simulink model "PassStFwdbkwdHolderChk"  (R2018b)
settings: Solver=FixedStepDiscrete  StartTime=0.0  StopTime=10.0  RelTol=1e-3
libraries: simulink x1
settings Model: Creator=sn2xws  LastModifiedBy=sn2xws
settings Model: ModifiedHistory=|
  | 2024.6.26 V3.0.0 557模式流程
  | 2024.11.18 V3.0.1 增加Md58 Retry
  | 2024.12.11 V3.0.2 Md57 Md58 反复retry的bug修复 BUG 960388 BUG 960408
  | 25.7.4 V3.13.0 新增Md61 Md62
settings DataIOCC: SaveFormat=StructureWithTime
settings OptimizationCC: DefaultParameterBehavior=Inlined  EnhancedBackFolding=on  PassReuseOutputArgsAs=Individual arguments  ZeroExternalMemoryAtStartup=off  ZeroInternalMemoryAtStartup=off  OptimizeBlockOrder=speed  DifferentSizesBufferReuse=on  OptimizationCustomize=off
settings DebuggingCC: ParameterTunabilityLossMsg=error
settings SFSimCC: MATLABDynamicMemAlloc=off
settings RTWCC: SystemTargetFile=autosar.tlc  GenCodeOnly=on  TemplateMakefile=ert_default_tmf  Description=AUTOSAR  GenerateReport=on  IncludeHyperlinkInReport=on  LaunchReport=on  GenerateTraceInfo=on  GenerateTraceReport=on  GenerateTraceReportSl=on  GenerateTraceReportSf=on  GenerateTraceReportEml=on
settings CodeAppCC: ForceParamTrailComments=on  IgnoreCustomStorageClasses=off  OperatorAnnotations=on  SimulinkDataObjDesc=on  SFDataObjDesc=on  InsertBlockDesc=on
settings STFCustomTargetCC: TargetLangStandard=C99 (ISO)  MultiwordLength=256  ParMdlRefBuildCompliant=on  CompOptLevelCompliant=on  IncludeMdlTerminateFcn=off  CombineOutputUpdateFcns=on  SuppressErrorStatus=on  ERTCustomFileBanners=on  SupportNonFinite=off  SupportComplex=off  SupportContinuousTime=off  SupportNonInlinedSFcns=off  RemoveResetFunc=on  MATLABClassNameForMDSCustomization=Simulink.SoftwareTarget.ERTCustomization  AutosarCompliant=on  UseToolchainInfoCompliant=on  LookupTableObjectStructAxisOrder=2,1,3,4,...  LUTObjectStructOrderEvenSpacing=Size,Table,Breakpoints  SystemTargetFile=autosar.tlc
settings ERTTargetCC: TargetLangStandard=C99 (ISO)  ConcurrentExecutionCompliant=off  IncludeMdlTerminateFcn=off  SuppressErrorStatus=on  SupportNonFinite=off  SupportComplex=off  ModelStepFunctionPrototypeControlCompliant=off  CPPClassGenCompliant=off  AutosarCompliant=on  LookupTableObjectStructAxisOrder=2,1,3,4,...  LUTObjectStructOrderEvenSpacing=Size,Table,Breakpoints  InlinedParameterPlacement=NonHierarchical  ERTCustomFileTemplate=example_file_process.tlc  ERTFilePackagingFormat=Compact

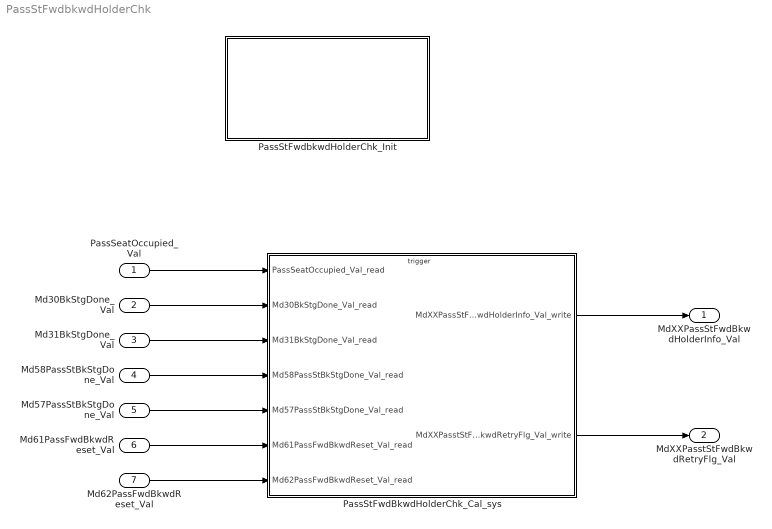
== system PassStFwdbkwdHolderChk ==
  PassSeatOccupied_Val : Inport  OutDataTypeStr=boolean  PortDimensions=1
  Md30BkStgDone_Val : Inport  Port=2  OutDataTypeStr=boolean  PortDimensions=1
  Md31BkStgDone_Val : Inport  Port=3  OutDataTypeStr=boolean  PortDimensions=1
  Md58PassStBkStgDone_Val : Inport  Port=4  OutDataTypeStr=boolean  PortDimensions=1
  Md57PassStBkStgDone_Val : Inport  Port=5  OutDataTypeStr=boolean  PortDimensions=1
  Md61PassFwdBkwdReset_Val : Inport  Port=6  OutDataTypeStr=boolean  PortDimensions=1
  Md62PassFwdBkwdReset_Val : Inport  Port=7  OutDataTypeStr=boolean  PortDimensions=1
  PassStFwdBkwdHolderChk_Cal_sys : Subsystem
  PassStFwdbkwdHolderChk_Init : Subsystem
  MdXXPassStFwdBkwdHolderInfo_Val : Outport  OutDataTypeStr=uint32  PortDimensions=1
  MdXXPasstStFwdBkwdRetryFlg_Val : Outport  Port=2  OutDataTypeStr=uint32  PortDimensions=1
  wires:
  PassSeatOccupied_Val/1 -> PassStFwdBkwdHolderChk_Cal_sys/1(PassSeatOccupied_Val_read)
  PassStFwdBkwdHolderChk_Cal_sys/1(MdXXPassStFwdBkwdHolderInfo_Val_write) -> MdXXPassStFwdBkwdHolderInfo_Val/1
  Md30BkStgDone_Val/1 -> PassStFwdBkwdHolderChk_Cal_sys/2(Md30BkStgDone_Val_read)
  Md31BkStgDone_Val/1 -> PassStFwdBkwdHolderChk_Cal_sys/3(Md31BkStgDone_Val_read)
  PassStFwdBkwdHolderChk_Cal_sys/2(MdXXPasstStFwdBkwdRetryFlg_Val_write) -> MdXXPasstStFwdBkwdRetryFlg_Val/1
  Md58PassStBkStgDone_Val/1 -> PassStFwdBkwdHolderChk_Cal_sys/4(Md58PassStBkStgDone_Val_read)
  Md57PassStBkStgDone_Val/1 -> PassStFwdBkwdHolderChk_Cal_sys/5(Md57PassStBkStgDone_Val_read)
  Md61PassFwdBkwdReset_Val/1 -> PassStFwdBkwdHolderChk_Cal_sys/6(Md61PassFwdBkwdReset_Val_read)
  Md62PassFwdBkwdReset_Val/1 -> PassStFwdBkwdHolderChk_Cal_sys/7(Md62PassFwdBkwdReset_Val_read)

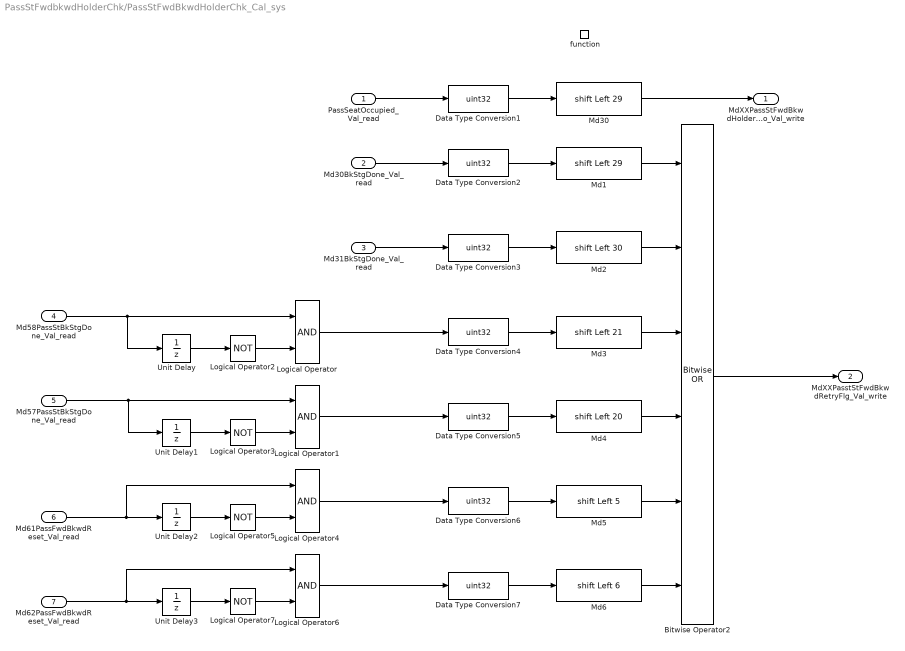
== system PassStFwdbkwdHolderChk/PassStFwdBkwdHolderChk_Cal_sys ==
  PassSeatOccupied_Val_read : Inport
  Md30BkStgDone_Val_read : Inport  Port=2
  Md31BkStgDone_Val_read : Inport  Port=3
  Md58PassStBkStgDone_Val_read : Inport  Port=4
  Md57PassStBkStgDone_Val_read : Inport  Port=5
  Md61PassFwdBkwdReset_Val_read : Inport  Port=6
  Md62PassFwdBkwdReset_Val_read : Inport  Port=7
  function : TriggerPort  TriggerType=function-call  IsSimulinkFunction=on  FunctionName=PassStFwdBkwdHolderChk_Cal  VariantControl=(inherit)
  Bitwise Operator2 : simulink/Logic and Bit Operations/Bitwise Operator  logicop=OR  UseBitMask=off  NumInputPorts=6  BitMask=bin2dec('11011001')  BitMaskRealWorld=Stored Integer
  Data Type Conversion{1..7} (7 alike) : DataTypeConversion  OutDataTypeStr=uint32
  Logical Operator{,1,4,6} (4 alike) : Logic  AllPortsSameDT=off  OutDataTypeStr=boolean
  Logical Operator{2..3,5,7} (4 alike) : Logic  Operator=NOT  Inputs=1  AllPortsSameDT=off  OutDataTypeStr=boolean
  Md1 : ArithShift  BitShiftNumber=29  BitShiftDirection=Left
  Md2 : ArithShift  BitShiftNumber=30  BitShiftDirection=Left
  Md3 : ArithShift  BitShiftNumber=21  BitShiftDirection=Left
  Md30 : ArithShift  BitShiftNumber=29  BitShiftDirection=Left
  Md4 : ArithShift  BitShiftNumber=20  BitShiftDirection=Left
  Md5 : ArithShift  BitShiftNumber=5  BitShiftDirection=Left
  Md6 : ArithShift  BitShiftNumber=6  BitShiftDirection=Left
  Unit Delay{,1..3} (4 alike) : UnitDelay  SampleTime=-1
  MdXXPassStFwdBkwdHolderInfo_Val_write : Outport
      settings: EnsureOutportIsVirtual=on
  MdXXPasstStFwdBkwdRetryFlg_Val_write : Outport  Port=2
      settings: EnsureOutportIsVirtual=on
  wires:
  PassSeatOccupied_Val_read/1 -> Data Type Conversion1/1
  Data Type Conversion1/1 -> Md30/1
  Md30/1 -> MdXXPassStFwdBkwdHolderInfo_Val_write/1
  Md30BkStgDone_Val_read/1 -> Data Type Conversion2/1
  Md31BkStgDone_Val_read/1 -> Data Type Conversion3/1
  Bitwise Operator2/1 -> MdXXPasstStFwdBkwdRetryFlg_Val_write/1
  Data Type Conversion2/1 -> Md1/1
  Data Type Conversion3/1 -> Md2/1
  Md1/1 -> Bitwise Operator2/1
  Md2/1 -> Bitwise Operator2/2
  Data Type Conversion4/1 -> Md3/1
  Md3/1 -> Bitwise Operator2/3
  Md4/1 -> Bitwise Operator2/4
  Data Type Conversion5/1 -> Md4/1
  Logical Operator/1 -> Data Type Conversion4/1
  Md58PassStBkStgDone_Val_read/1 -> Unit Delay/1, Logical Operator/1
  Logical Operator1/1 -> Data Type Conversion5/1
  Md57PassStBkStgDone_Val_read/1 -> Unit Delay1/1, Logical Operator1/1
  Logical Operator2/1 -> Logical Operator/2
  Unit Delay/1 -> Logical Operator2/1
  Logical Operator3/1 -> Logical Operator1/2
  Unit Delay1/1 -> Logical Operator3/1
  Data Type Conversion6/1 -> Md5/1
  Md5/1 -> Bitwise Operator2/5
  Md6/1 -> Bitwise Operator2/6
  Data Type Conversion7/1 -> Md6/1
  Unit Delay2/1 -> Logical Operator5/1
  Logical Operator5/1 -> Logical Operator4/2
  Md61PassFwdBkwdReset_Val_read/1 -> Logical Operator4/1, Unit Delay2/1
  Logical Operator4/1 -> Data Type Conversion6/1
  Logical Operator6/1 -> Data Type Conversion7/1
  Md62PassFwdBkwdReset_Val_read/1 -> Logical Operator6/1, Unit Delay3/1
  Logical Operator7/1 -> Logical Operator6/2
  Unit Delay3/1 -> Logical Operator7/1

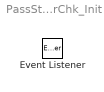
== system PassStFwdbkwdHolderChk/PassStFwdbkwdHolderChk_Init ==
  Event Listener : EventListener  EventName=reset
